simulink model "MATE_SynchronousMachineV2"  (R2024b)
settings: Solver=FixedStepDiscrete  StartTime=0.0  StopTime=6  FixedStep=Ts  RelTol=1e-4  EnableMultiTasking=on
PostLoadFcn:
  | Ts=25e-6;offset=4;
InitFcn:
  | Ts=25e-6;offset=4;
undefined symbols (not defined in the file): DiscIntNeverNeededParam, MATE, Phase, Rsnu, Single
libraries: fl_lib x76, nesl_utility x59, ee_lib x14, artemis x9, simetran x5, powerlib_extras x3, simetranss x2, simulink_extras x2, simulink x2
(part 2 of 5)

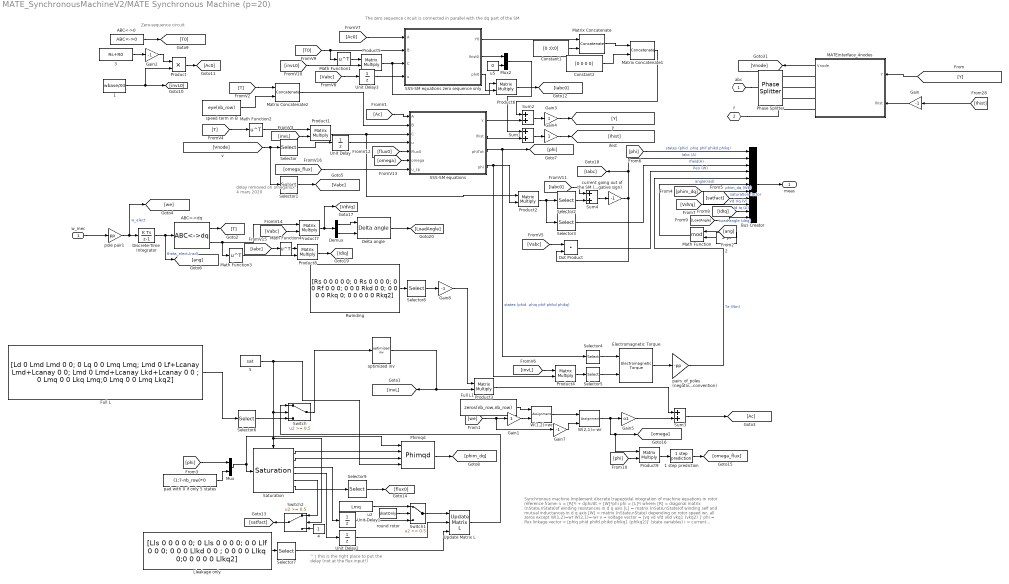
== system MATE_SynchronousMachineV2/MATE Synchronous Machine (p=20) ==
  note: delay removed
      | on omegaflux
      | 4 mars 2020
  note: Synchronous machine
      | Implement discrete trapezoidal integration of machine equations in rotor reference frame:
      |   v = [R]*i + dphi/dt + [W]*phi
      | phi = [L]*i
      |
      | where:
      | [R] = diagonal matrix (nState,nState)of winding resistances in d q axis
      | [L] = matrix (nSate,nState)of winding self and mutual inductances in d q axis
      | [W] = matrix (nState,nState) depending on rotor speed wr,
      |       all zeros except W(1,2)=wr  W(2,1)=-wr
      |
      |   v = voltage vector      = [vq   vd   vfd   vkd   vkq1   (vkq2)  ]'
      | phi = flux linkage vector = [phiq phid phifd phikd phikq1 (phikq2)]' (state variables)
      |   i = current vector      = [iq   id   ifd   ikd   ikq1   (ikq2)  ]'
      |
      | if RotorType=Salient-Pole, nState=5
      | if RotorType=Round,        nState=6
  note: ^
      | |
      | this is the right place to put the delay
      | (not at the flux input!)
  note: The zero sequence circuit is connected in parallel with the dq part of the SM
  note: Zero-sequence circuit
  w_mec : Inport
  1 : Constant  Value=wbase/X0
  1 step prediction : artemis/SSN/SSN rotating machines/SSN Synchronous Machine/1 step prediction  SystemSampleTime=-1  VariantActivationTime=update diagram  AllowFlexibleInterface=on  Latency=0  AutoFrameSizeCalculation=off
      settings: SourceProductName=Artemis
  2 : Constant  Value=2*pi
  3 : Constant  Value=Rs+R0
  4 : Constant
  5 : Constant  Value=sat
  ABC<->0 : artemis/SSN/SSN rotating machines/SSN Synchronous Machine/ABC<->0  SystemSampleTime=-1  VariantActivationTime=update diagram  AllowFlexibleInterface=on  Latency=0  AutoFrameSizeCalculation=off
      settings: SourceProductName=Artemis
  ABC<->dq : artemis/SSN/SSN rotating machines/SSN Synchronous Machine/ABC<->dq  SystemSampleTime=-1  VariantActivationTime=update diagram  AllowFlexibleInterface=on  Latency=0  AutoFrameSizeCalculation=off
      settings: SourceProductName=Artemis
  Bus Creator : BusCreator  Inputs=11
  Constant1 : Constant  Value=[0 ;0;0]  VectorParams1D=off
  Constant2 : Constant  Value=[0 0 0 0]  VectorParams1D=off
  Delta angle : artemis/SSN/SSN rotating machines/SSN Synchronous Machine/Delta angle  SystemSampleTime=-1  VariantActivationTime=update diagram  AllowFlexibleInterface=on  Latency=0  AutoFrameSizeCalculation=off
      settings: SourceProductName=Artemis
  Demux : Demux  Outputs=2
  Discrete-Time Integrator : DiscreteIntegrator  InitialCondition=theta_0  SampleTime=Ts  ICPrevOutput=DiscIntNeverNeededParam  ICPrevScaledInput=DiscIntNeverNeededParam
  Dot Product : DotProduct  OutDataTypeStr=Inherit: Inherit via internal rule
  Electromagnetic Torque : artemis/SSN/SSN rotating machines/SSN Synchronous Machine/Electromagnetic Torque  SystemSampleTime=-1  VariantActivationTime=update diagram  AllowFlexibleInterface=on  Latency=0  AutoFrameSizeCalculation=off
      settings: SourceProductName=Artemis
  Full L : Constant  Value="[Ld 0 Lmd Lmd 0 0; 0 Lq 0 0  Lmq Lmq; Lmd 0 Lf+Lcanay Lmd+Lcanay 0 0; Lmd 0 Lmd+Lcanay Lkd+Lcanay 0 0 ; 0 Lmq 0 0 Lkq Lmq;0 Lmq 0 0 Lmq Lkq2]"
  Full L1 : Constant  Value=zeros(nb_row,nb_row)
  Gain : Gain  Gain=-1
  Gain1 : Gain  SaturateOnIntegerOverflow=on  OutDataTypeStr=Inherit: Same as input  ParamDataTypeStr=Inherit: Same as input
  Gain2 : Gain  Gain=-1
  Gain3 : Gain
  Gain4 : Gain
  Gain5 : Gain  Gain=o1
  Gain7 : Gain  Gain=-1  SaturateOnIntegerOverflow=on  OutDataTypeStr=Inherit: Same as input  ParamDataTypeStr=Inherit: Same as input
  Gain8 : Gain  Gain=-1
  Lleakage only : Constant  Value="[Lls 0 0 0 0 0; 0 Lls 0 0  0 0; 0 0 Llf 0 0 0; 0 0 0 Llkd 0 0 ; 0 0 0 0 Llkq 0;0 0 0 0 0 Llkq2]"
  MATEinterface_4nodes : Subsystem
  Math Function : Math  Operator=mod  SignedPower=on
  Math Function{1..4} (4 alike) : Math  Operator=transpose  SignedPower=on
  Matrix Concatenate : Concatenate  Mode=Multidimensional array  ConcatenateDimension=2
  Matrix Concatenate1 : Concatenate  Mode=Multidimensional array
  Matrix Concatenate2 : Concatenate  Mode=Multidimensional array  ConcatenateDimension=2
  Mux : Mux  Inputs=2
  Mux2 : Mux  Inputs=2
  Phase Splitter : ee_lib/Connectors & References/Phase Splitter
  Phimqd : artemis/SSN/SSN rotating machines/SSN Synchronous Machine/Phimqd  SystemSampleTime=-1  VariantActivationTime=update diagram  AllowFlexibleInterface=on  Latency=0  AutoFrameSizeCalculation=off
      settings: SourceProductName=Artemis
  Product : Product  RndMeth=Zero
  Product{1..9} (9 alike) : Product  Multiplication=Matrix(*)  SaturateOnIntegerOverflow=on  OutDataTypeStr=Inherit: Same as first input
  Rwinding : Constant  Value="[Rs 0 0 0 0 0; 0 Rs 0 0 0 0; 0 0 Rf  0 0 0; 0 0 0 Rkd 0 0; 0 0 0 0  Rkq 0; 0 0 0 0 0 Rkq2]"
  SSS-SM equations : Subsystem
  SSS-SM equations zero sequence only : Subsystem
  Saturation : artemis/SSN/SSN rotating machines/SSN Synchronous Machine/Saturation  SystemSampleTime=-1  VariantActivationTime=update diagram  AllowFlexibleInterface=on  Latency=0  AutoFrameSizeCalculation=off
      settings: SourceProductName=Artemis
  Selector : Selector  InputPortWidth=4  IndexOptions=Index vector (dialog)  Indices=[1 2 3 4]  OutputSizes=1
  Selector1 : Selector  InputPortWidth=4  IndexOptions=Index vector (dialog)  Indices=[1 2 3 ]  OutputSizes=1
  Selector2 : Selector  InputPortWidth=4  IndexOptions=Index vector (dialog)  Indices=[1 2 3 ]  OutputSizes=1
  Selector3 : Selector  InputPortWidth=4  IndexOptions=Index vector (dialog)  Indices=[4 ]  OutputSizes=1
  Selector4 : Selector  InputPortWidth=nb_row  IndexOptions=Index vector (dialog)  Indices=[1 2]  OutputSizes=1
  Selector5 : Selector  InputPortWidth=nb_row  IndexOptions=Index vector (dialog)  Indices=[1 2]  OutputSizes=1
  Selector6 : Selector  NumberOfDimensions=2  InputPortWidth=3  IndexOptions=Index vector (dialog),Index vector (dialog)  Indices=[1:nb_row],[1:nb_row]  OutputSizes=1,1
  Selector7 : Selector  NumberOfDimensions=2  InputPortWidth=3  IndexOptions=Index vector (dialog),Index vector (dialog)  Indices=[1:nb_row],[1:nb_row]  OutputSizes=1,1
  Selector8 : Selector  NumberOfDimensions=2  InputPortWidth=3  IndexOptions=Index vector (dialog),Index vector (dialog)  Indices=[1:nb_row],[1:nb_row]  OutputSizes=1,1
  Selector9 : Selector  InputPortWidth=6  IndexOptions=Index vector (dialog)  Indices=[1:nb_row]  OutputSizes=1
  Sum{1..4} (4 alike) : Sum  SaturateOnIntegerOverflow=on
  Switch : Switch  Threshold=0.5  SaturateOnIntegerOverflow=off  InputSameDT=off
  Switch1 : Switch  Threshold=0.5  SaturateOnIntegerOverflow=off  InputSameDT=off
  Switch2 : Switch  Threshold=0.5  SaturateOnIntegerOverflow=off  InputSameDT=off
  Unit Delay : UnitDelay  SampleTime=Ts  HasFrameUpgradeWarning=on
  Unit Delay1 : UnitDelay  InitialCondition=Lmq  SampleTime=Ts  HasFrameUpgradeWarning=on
  Unit Delay2 : UnitDelay  InitialCondition=Lmd  SampleTime=Ts  HasFrameUpgradeWarning=on
  Unit Delay3 : UnitDelay  SampleTime=Ts  HasFrameUpgradeWarning=on
  Update Matrix L : artemis/SSN/SSN rotating machines/SSN Synchronous Machine/Update Matrix L  SystemSampleTime=-1  VariantActivationTime=update diagram  AllowFlexibleInterface=on  Latency=0  AutoFrameSizeCalculation=off
      settings: SourceProductName=Artemis
  W(1,2)=wr : Assignment  NumberOfDimensions=2  IndexOptions=Index vector (dialog),Index vector (dialog)  Indices=1,2  OutputSizes=1,1
  W(2,1)=-wr : Assignment  NumberOfDimensions=2  IndexOptions=Index vector (dialog),Index vector (dialog)  Indices=2,1  OutputSizes=1,1
  current going out of the SM (negative sign) : Gain  Gain=-1
  optimized inv : artemis/SSN/SSN rotating machines/SSN Synchronous Machine/optimized inv  SystemSampleTime=-1  VariantActivationTime=update diagram  AllowFlexibleInterface=on  Latency=0  AutoFrameSizeCalculation=off
      settings: SourceProductName=Artemis
  pad with 0 if only 5 states : Constant  Value=(1:7-nb_row)*0
  pairs_of_poles (negative sign for generator convention) : Gain  Gain=-pp
  pole pair1 : Gain  Gain=pp
  round rotor : Constant  Value=dsatOnly
  speed term in B : Constant  Value=eye(nb_row)  VectorParams1D=off
  u2 : Constant  Value=Lmq
  u5 : Constant  Value=0
  "abc   " : PMIOPort  Side=Right
  f : PMIOPort  Port=2  Side=Left
  meas : Outport  VectorParamsAs1DForOutWhenUnconnected=off
  wires:
  [Ihist] -> Gain/1
  Constant1/1 -> Matrix Concatenate/2
  Lleakage only/1 -> Selector7/1
  Delta angle/1 -> [LoadAngle]
  Gain7/1 -> W(2,1)=-wr/2
  Matrix Concatenate1/1 -> Sum2/1
  [phi] -> Product9/2
  W(1,2)=wr/1 -> W(2,1)=-wr/1
  Product2/1 -> Selector2/1, Selector3/1
  Selector2/1 -> Sum4/2
  Unit Delay/1 -> SSS-SM equations/4(u)
  [Vabc] -> Product7/2
  [invL] -> Product1/2
  [omega] -> SSS-SM equations/6(omega)
  SSS-SM equations zero sequence only/3(phi0) -> Product6/2
  ABC<->dq/1 -> [T]
  SSS-SM equations/1(Y) -> Sum2/2
  [Vabc] -> Unit Delay3/1
  w_mec/1 -> pole pair1/1
  3/1 -> Gain2/1
  [IdIq] -> Bus Creator/10  "Id Iq (A)"
  Selector3/1 -> Bus Creator/3  "Ifield(A)"
  Matrix Concatenate2/1 -> SSS-SM equations/2(B)
  [Iabc] -> Math Function4/1
  current going out of the SM (negative sign)/1 -> Dot Product/2, Bus Creator/2, [Iabc]  "Iabc (A)"
  [T] -> Matrix Concatenate2/1
  1/1 -> Product/2, [invL0]
  Saturation/1 -> Phimqd/2
  Math Function1/1 -> Product5/1
  speed term in B/1 -> Matrix Concatenate2/2
  u5/1 -> Mux2/2
  u2/1 -> Switch1/1
  Selector8/1 -> Gain8/1
  [VdVq] -> Bus Creator/9  "Vd Vq (V)"
  Selector9/1 -> [flux0]
  Product4/1 -> Selector5/1
  Math Function3/1 -> Product8/2
  pad with 0 if only 5 states/1 -> Mux/2
  2/1 -> Math Function/2
  Mux/1 -> Phimqd/1, Saturation/1
  Product/1 -> [Ac0]
  SSS-SM equations/2(Ihist) -> Sum1/2
  [Ac] -> SSS-SM equations/1(A)
  Product8/1 -> [IdIq]
  Dot Product/1 -> Bus Creator/4  "Peo (W)"
  [we] -> Gain7/1, Gain1/1
  Product6/1 -> [Iabc0]
  Switch1/1 -> Update Matrix L/1
  Rwinding/1 -> Selector8/1
  Gain3/1 -> [Y]
  [phi] -> Mux/1
  [invL0] -> Product5/2
  Sum2/1 -> Gain3/1
  optimized inv/1 -> [invL], Product3/2
  [Iabc0] -> Sum4/1
  [Ac0] -> SSS-SM equations zero sequence only/1(A)
  Selector6/1 -> Switch/3
  Gain1/1 -> W(1,2)=wr/2
  Selector1/1 -> [Vabc]
  1 step prediction/1 -> [omega_flux]
  ABC<->dq/2 -> Math Function3/1, Product7/1
  Mux2/1 -> Sum1/1
  SSS-SM equations/4(phi) -> Product4/2, Product2/2
  [satfact] -> Bus Creator/8  "saturation factor"
  Full L1/1 -> W(1,2)=wr/1
  Full L/1 -> Selector6/1
  Selector/1 -> Unit Delay/1
  Switch/1 -> optimized inv/1
  [Vabc] -> Dot Product/1
  W(2,1)=-wr/1 -> Gain5/1, [omega], Product9/1
  Demux/2 -> Delta angle/2
  Product5/1 -> SSS-SM equations zero sequence only/3(C), Product6/1
  5/1 -> Switch2/2, Saturation/Enable, Switch/2, Phimqd/4
  Saturation/4 -> Unit Delay2/1
  Gain5/1 -> Sum3/2
  pairs_of_poles (negative sign for generator convention)/1 -> Bus Creator/5  "Te (Nm)"
  Bus Creator/1 -> meas/1
  [Vnode] -> Selector/1, Selector1/1
  [T0] -> SSS-SM equations zero sequence only/2(B), Math Function1/1
  Sum1/1 -> Gain4/1
  SSS-SM equations zero sequence only/2(Ihist0) -> Mux2/1
  Gain2/1 -> Product/1
  Phimqd/1 -> [phim_dq]
  Unit Delay3/1 -> SSS-SM equations zero sequence only/4(u)
  SSS-SM equations zero sequence only/1(Y0) -> Matrix Concatenate/1
  [flux0] -> SSS-SM equations/5(Flux0)
  Demux/1 -> Delta angle/1
  Constant2/1 -> Matrix Concatenate1/2
  Gain8/1 -> Product3/1
  round rotor/1 -> Switch1/2
  Math Function2/1 -> Product1/1
  Switch2/1 -> [satfact]
  Update Matrix L/1 -> Switch/1
  Product1/1 -> SSS-SM equations/3(C), Product2/1
  SSS-SM equations/3(phiTot) -> Selector4/1, [phi]  "states (phid  phiq phif phikd phikq)"
  4/1 -> Switch2/3
  Sum3/1 -> [Ac]
  [T] -> Math Function2/1
  Selector7/1 -> Update Matrix L/3
  Product9/1 -> 1 step prediction/1
  Saturation/2 -> Phimqd/3
  Product3/1 -> Sum3/1
  Saturation/3 -> Unit Delay1/1
  Discrete-Time Integrator/1 -> [ang], ABC<->dq/1  "theta_elect (rad)"
  ABC<->0/1 -> [T0]
  Math Function/1 -> Bus Creator/6  "angle(rad)"
  pole pair1/1 -> Discrete-Time Integrator/1, [we]  "w_elect"
  Gain4/1 -> [Ihist]
  Unit Delay2/1 -> Update Matrix L/2
  Saturation/6 -> Selector9/1
  Electromagnetic Torque/1 -> pairs_of_poles (negative sign for generator convention)/1
  Math Function4/1 -> Product8/1
  [ang] -> Math Function/1
  [phi] -> Bus Creator/1  "states (phid  phiq phif phikd phikq)"
  Matrix Concatenate/1 -> Matrix Concatenate1/1
  [invL] -> Product4/1
  Unit Delay1/1 -> Switch1/3
  Selector4/1 -> Electromagnetic Torque/1
  Saturation/5 -> Switch2/1
  Product7/1 -> [VdVq], Demux/1
  [omega_flux] -> SSS-SM equations/7(u_sp)
  [phim_dq] -> Bus Creator/7  "phim_dq (Wb)"
  [LoadAngle] -> Bus Creator/11  "Load angle (deg)"
  Selector5/1 -> Electromagnetic Torque/2
  Sum4/1 -> current going out of the SM (negative sign)/1
  MATEinterface_4nodes/1(Vnode) -> [Vnode]
  [Y] -> MATEinterface_4nodes/1(Y)
  Gain/1 -> MATEinterface_4nodes/2(Ihist)
  connections:
  "abc   "/RConn1 -- Phase Splitter/LConn1
  MATEinterface_4nodes/RConn1 -- Phase Splitter/RConn1
  MATEinterface_4nodes/RConn2 -- Phase Splitter/RConn2
  MATEinterface_4nodes/RConn3 -- Phase Splitter/RConn3
  f/RConn1 -- MATEinterface_4nodes/RConn4

== system MATE_SynchronousMachineV2/MATE_LineCommutatedConverter ==
  g : Inport
  MATEPREP : Subsystem  Commented=on
  MATE_AGGREG : Subsystem
  Phase Splitter2 : ee_lib/Connectors & References/Phase Splitter
  abc : PMIOPort  Side=Left
  + : PMIOPort  Port=2  Side=Right
  - : PMIOPort  Port=3  Side=Right
  meas : Outport
  wires:
  g/1 -> MATEPREP/1(g), MATE_AGGREG/1(g)
  MATE_AGGREG/1(meas) -> meas/1
  connections:
  MATEPREP/RConn2 -- MATE_AGGREG/RConn2 -- -/RConn1
  MATEPREP/RConn1 -- MATE_AGGREG/RConn1 -- +/RConn1
  Phase Splitter2/RConn1 -- MATEPREP/LConn1 -- MATE_AGGREG/LConn1
  Phase Splitter2/RConn2 -- MATEPREP/LConn2 -- MATE_AGGREG/LConn2
  Phase Splitter2/RConn3 -- MATEPREP/LConn3 -- MATE_AGGREG/LConn3
  abc/RConn1 -- Phase Splitter2/LConn1

== system MATE_SynchronousMachineV2/Mesure et visualisation ==
  Discrete Mean value : Subsystem  mask(Discrete Mean value){Freq=60, Vinit=0, Ts=Ts}
      mask prompts: Freq "Fundamental frequency (Hz):"; Vinit "Initial input (DC component):"; Ts "Sample time:"
      mask help: Compute the mean value of the input signal over a running window of one cycle of the specified fundamental frequency.
      mask init:
      | SamplesPerCycle=1/Freq/Ts;
      | RoundSamplesPerCycle=ceil(SamplesPerCycle);
      | Delay=RoundSamplesPerCycle*Ts;
      | Corr1=(SamplesPerCycle-RoundSamplesPerCycle)/2;
      | Corr2=(SamplesPerCycle-RoundSamplesPerCycle)/SamplesPerCycle;
      | K1=Corr1*Corr2;
      | K2=Corr2 + Corr1*Corr2;
      mask Display: disp('Mean\n(discrete)')
  Mux : Mux  Inputs=2
  Mux3 : Mux  Inputs=2
  Mux4 : Mux  Inputs=2
  V1 Vref : Outport
  If IIfref : Outport  Port=2
  Vcc : Outport  Port=3
  wires:
  Discrete Mean value/1(Mean) -> Mux/2
  [Ucc] -> Mux/1, Discrete Mean value/1(In)
  Mux/1 -> Vcc/1  "Vcc - Vcc moyen (V)"
  [If] -> Mux3/1
  [Ifref] -> Mux3/2
  Mux3/1 -> If IIfref/1
  [V1] -> Mux4/1
  [Vref] -> Mux4/2
  Mux4/1 -> V1 Vref/1

== system MATE_SynchronousMachineV2/Model Initialization ==

== system MATE_SynchronousMachineV2/PQ ==
  note: 1) P = Va*Ia + Vb*Ib + Vc*Ic
  note: 2) Q = 1/sqrt(3)* (Vbc*Ia + Vca*Ib + Vab*Ic)
  note: This block computes the 3-phase instantaneous real power and reactive power using the following equations:
  note: Note: Equation 2 is valid only for a balanced and harmonic-free system.
  Vabc : Inport  PortDimensions=3
  Iabc : Inport  Port=2  PortDimensions=3
  Demux : Demux  Outputs=3
      settings: DisplayOption=none
  Mux : Mux  Inputs=3
  Mux1 : Mux  Inputs=2
  Product1 : Product  InputSameDT=on  SaturateOnIntegerOverflow=on  OutDataTypeStr=Inherit: Same as first input
  Product3 : Product  InputSameDT=on  SaturateOnIntegerOverflow=on  OutDataTypeStr=Inherit: Same as first input
  Sum : Sum  Inputs=+-  InputSameDT=on  SaturateOnIntegerOverflow=on  OutDataTypeStr=Inherit: Same as first input
  Sum1 : Sum  Inputs=1  InputSameDT=on  SaturateOnIntegerOverflow=on  OutDataTypeStr=Inherit: Same as first input
  Sum4 : Sum  Inputs=1  InputSameDT=on  SaturateOnIntegerOverflow=on  OutDataTypeStr=Inherit: Same as first input
  Sum5 : Sum  Inputs=+-  InputSameDT=on  SaturateOnIntegerOverflow=on  OutDataTypeStr=Inherit: Same as first input
  Sum6 : Sum  Inputs=+-  InputSameDT=on  SaturateOnIntegerOverflow=on  OutDataTypeStr=Inherit: Same as first input
  pu->V : Gain  Gain=1/sqrt(3)  SaturateOnIntegerOverflow=on  OutDataTypeStr=Inherit: Same as input  ParamDataTypeStr=Inherit: Same as input
  PQ : Outport  VectorParamsAs1DForOutWhenUnconnected=off
  wires:
  Sum1/1 -> pu->V/1
  Product3/1 -> Sum1/1
  Product1/1 -> Sum4/1
  Vabc/1 -> Product1/1, Demux/1
  Iabc/1 -> Product1/2, Product3/2
  Sum4/1 -> Mux1/1  "P"
  Demux/1 -> Sum/1, Sum6/2
  Demux/2 -> Sum/2, Sum5/1
  Demux/3 -> Sum5/2, Sum6/1
  Sum/1 -> Mux/3
  Sum5/1 -> Mux/1
  Sum6/1 -> Mux/2
  Mux/1 -> Product3/1
  pu->V/1 -> Mux1/2  "Q"
  Mux1/1 -> PQ/1

== system MATE_SynchronousMachineV2/turbine1 ==
  feild : Inport
  Te : Inport  Port=2
  Peo : Inport  Port=3
  Gain : Gain  Gain=1/(2*pi*60/20)
  Gain1 : Gain  Gain=1/202e6
  Gain3 : Gain  Gain=202e6
  Gain4 : Gain  Gain=1/(2*pi*60/20)
  Hydraulic Turbine and Governor : Subsystem  mask(Hydraulic Turbine and Governor){sm=[ 10/3  0.07 ], gate=[  0.01  0.97518  -0.1  0.1 ], reg=[  0.05  1.163  0.105  0  0.01  ], hyd=[  0  2.67  ], dref=0, po=0.802}
      mask prompts: sm "Servo-motor [ Ka()  Ta(sec) ]:"; gate "Gate opening limits [ gmin,gmax(pu)    vgmin,vgmax(pu/s) ]:"; reg "Permanent droop and regulator  [ Rp() Kp() Ki() Kd() Td(s) ]:"; hyd "Hydraulic turbine [ beta()  Tw(sec) ]:"; dref "Droop reference (0=power error, 1=gate opening):"; po "Initial mechanical power (pu):"
      mask help: Implements a hydraulic turbine combined to a PID governor system.
      mask init:
      | %block = gcb;
      | %[Ts, WantBlockChoice,ka,ta,gmin,gmax,vgmin,vgmax,Rp,Kp,ki,kd,td,beta,tw,go] = powericon('HydraulicTurbineInit',block,sm,gate,reg,hyd,po);
      | ka =sm (1 ); 
      | ta =sm (2 ); 
      | gmin =gate (1 ); 
      | gmax =gate (2 ); 
      | vgmin =gate (3 ); 
      | vgmax =gate (4 ); 
      | Rp =reg (1 ); 
      | kp =reg (2 ); 
      | ki =reg (3 ); 
      | kd =reg (4 ); 
      | td =reg (5 ); 
      | beta =hyd (1 ); 
      | tw =hyd (2 ); 
      | go =po *(gmax -gmin ); 
      | %powericon('SetInternalModels','set',block,WantBlockChoice);
      settings: OpenFcn=sps_rtmsupport('OpenFcn',gcbh)
      mask Help: helpview(psbhelp);
      mask Display: disp('')
  Mechanical model : Subsystem  mask(Synchronous machine mechanical model){J=3.4111e+06, F=0, fo=60/20, Ts=Ts}
      mask prompts: J "Inertia (kg.m^2)"; F "Friction (N.n.s)"; fo "Initial mechanical frequency (Hz)"; Ts "Sample Time (s)"
      mask help:
      | This is the mechanical equation of a synchronous machine.
      |
      | all values in SI.
      | J: inertia
      | F:friction
      | Te: torque input from the SM
      | Pin: power from the turbine
      | wmec: mechanical speed of the SM.
      | delta_wm: speed deviation
  Pref : Constant  Value=0.8
  Product1 : Product
  Terminator : Terminator
  wref : Constant
  w : Outport
  wires:
  Hydraulic Turbine and Governor/2(gate) -> Terminator/1
  Hydraulic Turbine and Governor/1(Pm) -> Gain3/1
  Gain1/1 -> Hydraulic Turbine and Governor/4(Pe0)
  Gain/1 -> Hydraulic Turbine and Governor/3(we)
  wref/1 -> Hydraulic Turbine and Governor/1(wref)
  Mechanical model/2(delta_wm) -> Gain4/1
  Pref/1 -> Product1/2
  Product1/1 -> Hydraulic Turbine and Governor/2(Pref)
  Gain3/1 -> Mechanical model/2(Pin)
  Mechanical model/1(wmec) -> Gain/1, w/1
  Gain4/1 -> Hydraulic Turbine and Governor/5(dw)
  feild/1 -> Product1/1
  Te/1 -> Mechanical model/1(Te)
  Peo/1 -> Gain1/1

== system MATE_SynchronousMachineV2/Command/Regulateur de courant ==
  If (pu) : Inport
  If_ref : Inport  Port=2
  Discrete 1st-Order Filter : Subsystem  mask(Discrete 1st-Order Filter){FilterType=Lowpass, Tc=1e-3, Ts=Ts, Initialize=off, Vac_Init=[0, 0, 60], Vdc_Init=0, PlotResponse=off, param1=[1 500 0.1]}
      mask prompts: FilterType "Filter Type:"; Tc "Time constant (s):"; Ts "Sample time:"; Initialize "Initialize filter states"; Vac_Init "AC initial input: [ Mag  Phase(degrees)  Freq(Hz) ]"; Vdc_Init "DC Initial input:"; PlotResponse "Plot filter response"; param1 "Frequency range(Hz) : [Start  End  Inc.]"
      mask init:
      | switch FilterType
      | case 1, % Lowpass
      |     X=[0 1 2 3 4];
      |     Y=[-2 -2 -3 -4 -4];
      |     numc=1;
      |     denc=[Tc 1];
      | case 2,   % Highpass
      |     X=[0 1 2 3 4];
      |     Y=[-4 -4 -3 -2 -2];
      |     numc=[1 0];
      |     denc=[1 1/Tc];
      | end
      | %
      | [Ac,Bc,Cc,Dc]=tf2ss(numc,denc);
      | %
      | %  Conversion to discrete transfer function
      | nstates = size(Ac,1);
      | if Ts<=0
      |     message = 'The Sample time parameter must be greater than zero. Note that specifying inherited sample time (-1) does not work for this block';
      |     error(message);
      | end
      | invexp = inv(eye(nstates) - (Ts/2)*Ac);
      | Ad = invexp*(eye(nstates) + (Ts/2)*Ac);
      | Bd = invexp*Bc;
      | Cd = Cc*invexp*Ts;
      | Dd = Cc*invexp*Bc*(Ts/2) + Dc;
      | %
      | if Initialize==1  % Compute initial conditions on states
      |     u1=Vac_Init(1)*exp(j*Vac_Init(2)*pi/180);
      |     u2=Vdc_Init*exp(j*90*pi/180);
      |     u=u1+u2;
      |     u0=imag(u); % input at  t=0;
      |     I=eye(size(Ac));
      |     sI1=I*j*(2*pi*Vac_Init(3));
      |     sI2=I*j*0;
      |     x=inv(sI1-Ac)*Bc*u1 + inv(sI2-Ac)*Bc*u2;
      |     x0c=imag(x);
      |     x0d=(I-Ac*Ts/2)*x0c/Ts - Bc/2*u0;
      | else
      |     x0d=0;
      | end
      | 
      | %
      | if PlotResponse==1 % Plot frequency and step response
      | t=[0:Tc/1000:7*Tc];
      | f=param1(1):param1(3):param1(2);
      | w=2*pi*f;
      | switch FilterType
      | 	case 1, % Lowpass
      | 		Ystep=1 - exp(-t/Tc);
      | 		RepFreq=1./(1+Tc*j.*w);
      | 	case 2,   % Highpass
      | 		Ystep=exp(-t/Tc);
      | 		RepFreq=1./(1 + (1./(Tc*j.*w)));
      | end
      | %
      | Mag=abs(RepFreq);
      | Pha=angle(RepFreq)*180/pi;
      | %
      | figure(1)
      | subplot(2,1,1)
      | plot(f,Mag)
      | grid
      | title('Bode Diagram')
      | ylabel('Magnitude')
      | subplot(2,1,2)
      | plot(f,Pha)
      | ylabel('Phase (deg)')
      | xlabel('Frequency (Hz)')
      | grid
      | figure(2)
      | plot(t,Ystep)
      | grid
      | ylabel('Amplitude')
      | xlabel('Time (s)')
      | title('Step Response')
      | end
      mask TypeOptions FilterType: Lowpass | Highpass
      mask Display: plot(X,Y);
  Discrete PI Controller1 : Subsystem  mask(Discrete PI Controller){Kp=400, Ki=1000, Par_Limits=[150 10], Init=79, Ts=Ts}
      mask prompts: Kp "Proportional gain (Kp):"; Ki "Integral gain (Ki):"; Par_Limits "Output limits: [ Upper   Lower ]"; Init "Output initial value:"; Ts "Sample time:"
      mask help: This block implements a basic discrete PI controller.
      mask init:
      | UpperLimit=Par_Limits(1);
      | LowerLimit=Par_Limits(2);
      mask Display: disp('PI');
  Sum : Sum  Inputs=|+-
  alpha : Outport
  wires:
  Discrete 1st-Order Filter/1(Out) -> Sum/1
  If (pu)/1 -> Discrete 1st-Order Filter/1(In)
  If_ref/1 -> Sum/2
  Sum/1 -> Discrete PI Controller1/1(Error)
  Discrete PI Controller1/1(Out) -> alpha/1

== system MATE_SynchronousMachineV2/Command/Regulateur de tension (Mode automatique) ==
  note: Regulateur de tension
  Vabc (pu) : Inport
  Vref : Inport  Port=2
  Discrete PI Controller1 : Subsystem  mask(Discrete PI Controller){Kp=Kp_V, Ki=Ki_V, Par_Limits=[2.46 0.33], Init=1, Ts=Ts}
      mask prompts: Kp "Proportional gain (Kp):"; Ki "Integral gain (Ki):"; Par_Limits "Output limits: [ Upper   Lower ]"; Init "Output initial value:"; Ts "Sample time:"
      mask help: This block implements a basic discrete PI controller.
      mask init:
      | UpperLimit=Par_Limits(1);
      | LowerLimit=Par_Limits(2);
      mask Display: disp('PI');
  Discrete 3-phase Positive-Sequence Fundamental Value : Subsystem  mask(Discrete 3-phase Positive-sequence fundamental value){Freq=60, Par_Init=[0 0], Ts=Ts}
      mask prompts: Freq "Fundamental frequency (Hz):"; Par_Init "Initial input (positive component): [ Mag  Phase(degrees) ]"; Ts "Sample time:"
      mask help: Compute the positive-sequence component of the input signal at the given fundamental frequency. The input is set of three balanced or unbalanced signals which may contain harmonics.
      mask init:
      | SamplesPerCycle=1/Freq/Ts;
      | RoundSamplesPerCycle=round(SamplesPerCycle);
      | Delay=RoundSamplesPerCycle*Ts - Ts/2;
      | Correction=SamplesPerCycle/RoundSamplesPerCycle - 1;
      | Real_Init=Par_Init(1)*cos(pi/180*Par_Init(2));
      | Imag_Init=Par_Init(1)*sin(pi/180*Par_Init(2));
      mask Display: disp('')
  Sum : Sum  Inputs=|-+
  Terminator : Terminator
  Iref : Outport
  tag scope: V1=global, Vref=global
  wires:
  Discrete 3-phase Positive-Sequence Fundamental Value/2(Phase) -> Terminator/1
  Vabc (pu)/1 -> Discrete 3-phase Positive-Sequence Fundamental Value/1(abc)
  Discrete PI Controller1/1(Out) -> Iref/1
  Sum/1 -> Discrete PI Controller1/1(Error)
  Vref/1 -> Sum/2, [Vref]
  Discrete 3-phase Positive-Sequence Fundamental Value/1(Mag) -> Sum/1, [V1]

== system MATE_SynchronousMachineV2/Command/Synchro Generateur d'mpulsions  ==
  Vabc_138 (pu) : Inport
  alpha(deg) : Inport  Port=2
  Demux : Demux  Outputs=3
  Discrete 3-phase PLL : Subsystem  mask(Discrete 3-phase PLL){Fmin=45, Par_Init=[0 60], ParK=[ 180 3200 1 ], Ts=Ts, AGC=on}
      mask prompts: Fmin "Minimum frequency (Hz):"; Par_Init "Initial inputs:[ Phase(degrees)   Frequency(Hz) ]"; ParK "Regulator gains [ Kp  Ki  Kd ]"; Ts "Sample time:"; AGC "Enable Automatic Gain Control"
      mask help:
      | This Phase Locked Loop (PLL) system can be used  to synchronize on a set of variable frequency, three-phase sinusoidal signals. If the Automatic Gain Control is enabled, the input (phase error) of the PLL regulator is scaled according to the input signals magnitude.
      |
      | For optimal performance, the following settings are recommended:
      |   [ Kp Ki  Kd ] = [ 180  3200  1 ]
      |   "Enable Automatic Gain Control" checked
      |
      | Input 1: Vector containing the normalized three-phase signals [Va Vb Vc]
      | Output 1:  Measured frequency (Hz) = w/(2pi)
      | Output 2:  Ramp w.t varying between  0 and 2*pi,
      |      synchronized on zero crossings of the fundamental (positive-sequence) of phase A.
      | Output 3: Vector [sin(wt) cos(wt)]
      mask init:
      | Kp=ParK(1);
      | Ki=ParK(2);
      | if length(ParK)==2
      |     Kd=0;
      | else
      |     Kd=ParK(3);
      | end    
      | Phase_Init=Par_Init(1);
      | Finit=Par_Init(2);
      settings: OpenFcn=power_openblockproxy();
      mask Display: disp('')
  Discrete Synchronized 12-Pulse Generator : Subsystem  mask(Discrete synchronized 12-pulse generator){Delta=D1 (lagging), pwidth=20, Double_Pulse=on, Ts=Ts}
      mask prompts: Delta "Delta winding connection"; pwidth "Pulse width (degrees)"; Double_Pulse "Double pulsing"; Ts "Sample time"
      mask help:
      | Use this block to fire the 12 thyristors of a 12-pulse converter.
      | Outputs 1 and 2 are two vectors of 6 pulses (0-1) to be sent to the two 6-pulse half bridges connected respectively to the Wye(Y) and Delta (D1 or D11) connected windings of the YYD converter transformer.
      | Pulses are individually synchronized on the 6 commutation voltages and generated alpha degrees after the increasing zero-crossings of the commutation voltages. The D pulses are either lagging or leading the Y pulses by 30 degrees.
      |
      | Input 'alpha_deg' :  Alpha firing signal (degrees).
      | Inputs 'A,B,C' : Phase-to-ground synchronization voltages  measured at the  primary side of the converter transformer.
      | Input 'Freq' : Frequency of the synchronization voltages (use a constant or the Freq PLL output)
      | Input 'Block' allows  blocking of the pulses when the applied signal is non zero.
      |
      | When the 'Douple pulsing' option is checked, two pulses are sent to each thyristor: a 1st pulse when the alpha angle is reached, then a 2nd pulse 60 degrees later, when the next thyristor is fired.
      mask init:
      | if (Delta == 1)
      |     D1 = 1;
      | else
      |     D1 = 0;
      | end
      mask TypeOptions Delta: D1 (lagging) | D11 (leading)
      mask Display: plot(0,0,100,100,[80 62 62 47 47 30],[40 40 60 60 40 40]-5)
  Ground2 : Ground
  Terminator : Terminator
  Terminator1 : Terminator
  Terminator2 : Terminator
  P : Outport
  wires:
  Vabc_138 (pu)/1 -> Discrete 3-phase PLL/1(Vabc(pu)), Demux/1
  Ground2/1 -> Discrete Synchronized 12-Pulse Generator/6(Block)
  alpha(deg)/1 -> Discrete Synchronized 12-Pulse Generator/1(alpha_deg)
  Demux/1 -> Discrete Synchronized 12-Pulse Generator/2(A)
  Demux/2 -> Discrete Synchronized 12-Pulse Generator/3(B)
  Demux/3 -> Discrete Synchronized 12-Pulse Generator/4(C)
  Discrete 3-phase PLL/1(Freq) -> Discrete Synchronized 12-Pulse Generator/5(Freq)
  Discrete Synchronized 12-Pulse Generator/2(PD) -> P/1
  Discrete 3-phase PLL/2(wt) -> Terminator/1
  Discrete 3-phase PLL/3(Sin_Cos) -> Terminator1/1
  Discrete Synchronized 12-Pulse Generator/1(PY) -> Terminator2/1

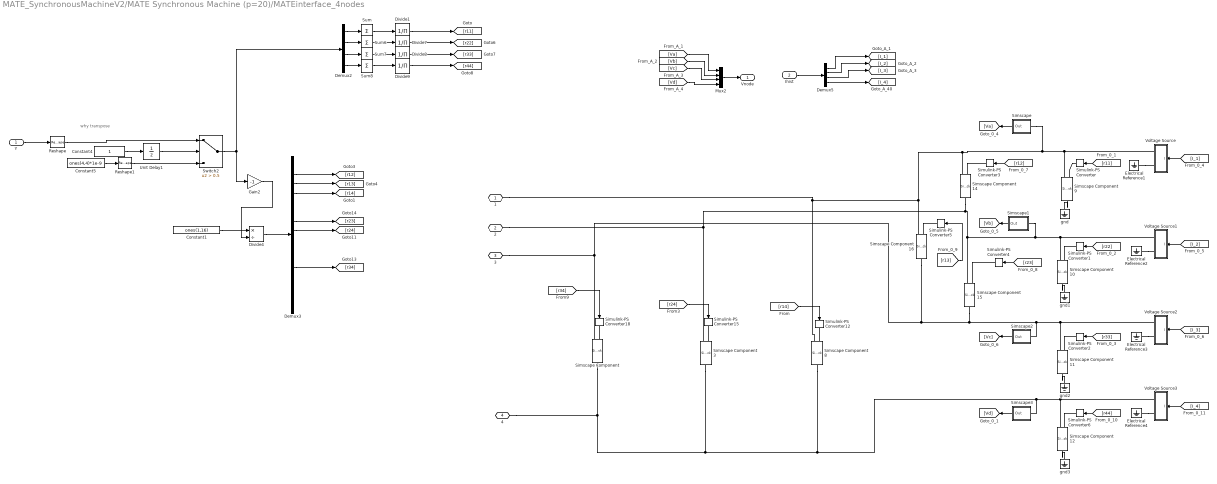
== system MATE_SynchronousMachineV2/MATE Synchronous Machine (p=20)/MATEinterface_4nodes ==
  note: why transpose
  Y : Inport
  Ihist : Inport  Port=2
  Constant1 : Constant  Value=ones(1,16)
  Constant4 : Constant
  Constant5 : Constant  Value=ones(4,4)*1e-9
  Demux2 : Demux  Outputs=[4 4 4 4]
      settings: DisplayOption=none
  Demux3 : Demux  Outputs=16
      settings: DisplayOption=none
  Demux5 : Demux  Outputs=[1 1 1 1 ]
      settings: DisplayOption=none
  Divide{1,7..9} (4 alike) : Product  Inputs=/
  Divide4 : Product  Inputs=*/  CollapseMode=Specified dimension
  Electrical Reference{1..4} (4 alike) : fl_lib/Electrical/Electrical Elements/Electrical Reference
  Gain2 : Gain  Gain=-1
  Mux2 : Mux  Inputs=[1 1 1 1 ]
  Reshape : Reshape
  Reshape1 : Reshape
  Simscape : Subsystem
      mask Display: disp('V')
  Simscape Component{,3,8..12,14..16} (10 alike) : SimscapeComponentBlock  SourceFile=variable_resistor_unlimited  ComponentPath=variable_resistor_unlimited  ComponentVariants="[\"variable_resistor_unlimited\"]"  ComponentVariantNames="[\"variable_resistor_unlimited\"]"  ClassName=variable_resistor_unlimited  SchemaVersion=1  R0=0 Ohm  Rmaxp=1e9 Ohm  Rmaxn=-1e9 Ohm  Rminp=1e-9 Ohm  Rminn=-1e-9 Ohm  i_specify=off  i_priority=None  i=0 A  i_nominal_specify=off  i_nominal_value=1  i_nominal_unit=A  v_specify=off  v_priority=None  v=0 V  v_nominal_specify=off  v_nominal_value=1  v_nominal_unit=V
      settings: CopyFcn=simscape.engine.sli.internal.componentblockcallback(gcbh,'COPY')  PreCopyFcn=simscape.engine.sli.internal.componentblockcallback(gcbh,'PRECOPY')  PreDeleteFcn=simscape.engine.sli.internal.componentblockcallback(gcbh,'PREDELETE')  InternalSimscapePortConfiguration="{\"Bottom\":[],\"Left\":[{\"id\":\"R\",\"label\":\"R\",\"type\":\"input\"},{\"id\":\"p\",\"label\":\"+\",\"type\":\"foundation.electrical.electrical\"}],\"Right\":[{\"id\":\"n\",\"label\":\"-\",\"type\":\"foundation.electrical.electrical\"}],\"Top\":[]}"
      mask Type: Variable Resistor
  Simscape1 : Subsystem
      mask Display: disp('V')
  Simscape2 : Subsystem
      mask Display: disp('V')
  Simscape3 : Subsystem
      mask Display: disp('V')
  Simulink-PS Converter{,1..6,12,15,18} (10 alike) : nesl_utility/Simulink-PS Converter  PhysicalDomain=network_engine_domain  SubClassName=ps_input  LeftPortType=input  RightPortType=output  PseudoPeriodic=off  Frequencies=[]  NoiseDistribution=none  NoiseParameters=[]  Unit=1  AffineConversion=off  FilteringAndDerivatives=provide  SimscapeFilterOrder=1  InputFilterTimeConstant=0.001  UdotUserProvided=0
  Sum{,6..8} (4 alike) : Sum  Inputs=+
  Switch2 : Switch  Criteria=u2 > Threshold  Threshold=0.5  SaturateOnIntegerOverflow=off  InputSameDT=off
  Unit Delay1 : UnitDelay  SampleTime=Ts  HasFrameUpgradeWarning=on
  Voltage Source : Subsystem
  Voltage Source1 : Subsystem
  Voltage Source2 : Subsystem
  Voltage Source3 : Subsystem
  gnd{,1..3} (4 alike) : fl_lib/Electrical/Electrical Elements/Electrical Reference
  1 : PMIOPort  Side=Right
  2 : PMIOPort  Port=2  Side=Right
  3 : PMIOPort  Port=3  Side=Right
  4 : PMIOPort  Port=4  Side=Right
  Vnode : Outport  VectorParamsAs1DForOutWhenUnconnected=off
  wires:
  [I_2] -> Voltage Source1/1(I)
  Simscape2/1(Out) -> [Vc]
  [I_3] -> Voltage Source2/1(I)
  Simscape/1(Out) -> [Va]
  Simscape1/1(Out) -> [Vb]
  [I_1] -> Voltage Source/1(I)
  Y/1 -> Reshape/1
  [r11] -> Simulink-PS Converter/1
  Sum/1 -> Divide1/1
  Divide1/1 -> [r11]
  [r22] -> Simulink-PS Converter1/1
  [r33] -> Simulink-PS Converter2/1
  [r12] -> Simulink-PS Converter3/1
  [r23] -> Simulink-PS Converter4/1
  [r13] -> Simulink-PS Converter5/1
  Demux2/1 -> Sum/1
  Divide7/1 -> [r22]
  Sum6/1 -> Divide7/1
  Demux2/2 -> Sum6/1
  Sum7/1 -> Divide8/1
  Divide8/1 -> [r33]
  Demux2/3 -> Sum7/1
  Demux2/4 -> Sum8/1
  Divide9/1 -> [r44]
  Sum8/1 -> Divide9/1
  [r44] -> Simulink-PS Converter6/1
  [I_4] -> Voltage Source3/1(I)
  Simscape3/1(Out) -> [Vd]
  [r14] -> Simulink-PS Converter12/1
  [r24] -> Simulink-PS Converter15/1
  Mux2/1 -> Vnode/1
  Ihist/1 -> Demux5/1
  Demux3/2 -> [r12]
  Demux3/3 -> [r13]
  Demux3/4 -> [r14]
  Constant1/1 -> Divide4/1
  [r34] -> Simulink-PS Converter18/1
  Reshape/1 -> Switch2/1
  Unit Delay1/1 -> Switch2/2
  Constant4/1 -> Unit Delay1/1
  Reshape1/1 -> Switch2/3
  Gain2/1 -> Divide4/2
  Demux5/4 -> [I_4]
  Demux5/3 -> [I_3]
  Demux5/2 -> [I_2]
  Demux5/1 -> [I_1]
  [Vd] -> Mux2/4
  [Vc] -> Mux2/3
  [Vb] -> Mux2/2
  [Va] -> Mux2/1
  Constant5/1 -> Reshape1/1
  Switch2/1 -> Demux2/1, Gain2/1
  Divide4/1 -> Demux3/1
  Demux3/7 -> [r23]
  Demux3/8 -> [r24]
  Demux3/12 -> [r34]
  connections:
  Simscape Component14/LConn2 -- Simscape Component9/LConn2 -- Voltage Source/RConn1 -- Simscape/LConn1 -- Simscape Component16/LConn2 -- 1/RConn1 -- Simscape Component8/LConn2
  Simscape Component11/LConn2 -- Voltage Source2/RConn1 -- Simscape2/LConn1 -- Simscape Component15/RConn1 -- Simscape Component16/RConn1 -- Simscape Component/LConn2 -- 3/RConn1
  Simscape Component10/LConn2 -- Voltage Source1/RConn1 -- Simscape1/LConn1 -- Simscape Component15/LConn2 -- Simscape Component14/RConn1 -- Simscape Component3/LConn2 -- 2/RConn1
  Electrical Reference2/LConn1 -- Voltage Source1/RConn2
  Electrical Reference3/LConn1 -- Voltage Source2/RConn2
  Electrical Reference1/LConn1 -- Voltage Source/RConn2
  Simscape Component9/RConn1 -- gnd/LConn1
  Simscape Component9/LConn1 -- Simulink-PS Converter/RConn1
  Simscape Component10/RConn1 -- gnd1/LConn1
  Simscape Component10/LConn1 -- Simulink-PS Converter1/RConn1
  Simscape Component11/RConn1 -- gnd2/LConn1
  Simscape Component11/LConn1 -- Simulink-PS Converter2/RConn1
  Simscape Component14/LConn1 -- Simulink-PS Converter3/RConn1
  Simscape Component15/LConn1 -- Simulink-PS Converter4/RConn1
  Simscape Component16/LConn1 -- Simulink-PS Converter5/RConn1
  4/RConn1 -- Simscape Component/RConn1 -- Simscape Component3/RConn1 -- Simscape Component8/RConn1 -- Simscape Component12/LConn2 -- Voltage Source3/RConn1 -- Simscape3/LConn1
  Simscape Component12/LConn1 -- Simulink-PS Converter6/RConn1
  Simscape Component12/RConn1 -- gnd3/LConn1
  Electrical Reference4/LConn1 -- Voltage Source3/RConn2
  Simscape Component8/LConn1 -- Simulink-PS Converter12/RConn1
  Simscape Component3/LConn1 -- Simulink-PS Converter15/RConn1
  Simscape Component/LConn1 -- Simulink-PS Converter18/RConn1

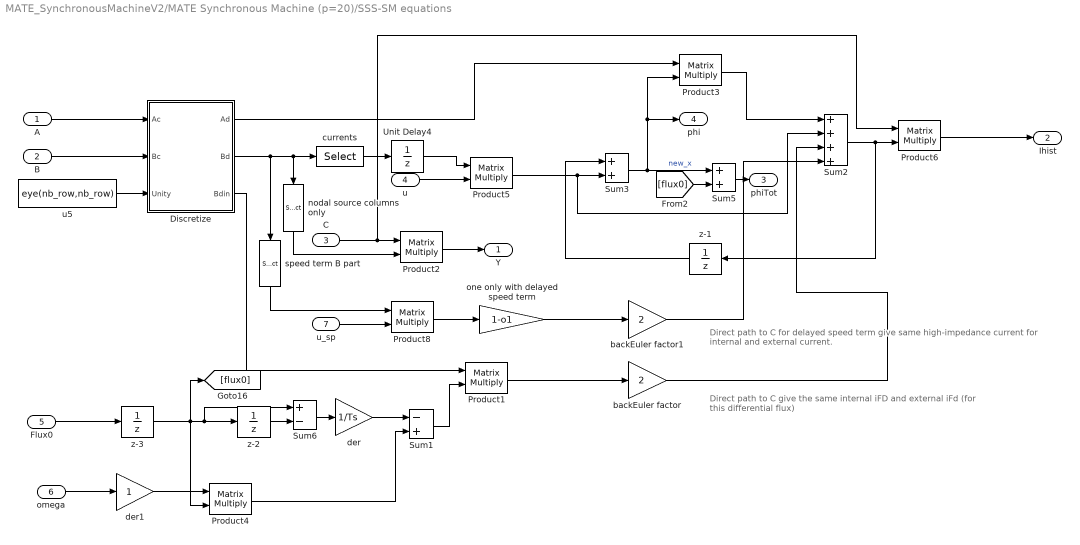
== system MATE_SynchronousMachineV2/MATE Synchronous Machine (p=20)/SSS-SM equations ==
  note: Direct path to C for delayed speed term give same high-impedance current
      | for internal and external current.
  note: Direct path to C give the same internal iFD and external iFd
      | (for this differential flux)
  A : Inport
  B : Inport  Port=2
  C : Inport  Port=3
  u : Inport  Port=4
  Flux0 : Inport  Port=5
  omega : Inport  Port=6
  u_sp : Inport  Port=7
  Discretize : Subsystem
  Product{1..6,8} (7 alike) : Product  Multiplication=Matrix(*)  SaturateOnIntegerOverflow=on  OutDataTypeStr=Inherit: Same as first input
  Sum1 : Sum  Inputs=-+  SaturateOnIntegerOverflow=on
  Sum2 : Sum  Inputs=++++  SaturateOnIntegerOverflow=on
  Sum3 : Sum  SaturateOnIntegerOverflow=on
  Sum5 : Sum  SaturateOnIntegerOverflow=on
  Sum6 : Sum  Inputs=+-  SaturateOnIntegerOverflow=on
  Unit Delay4 : UnitDelay  SampleTime=Ts  HasFrameUpgradeWarning=on
  backEuler factor : Gain  Gain=2  SaturateOnIntegerOverflow=on  OutDataTypeStr=Inherit: Same as input  ParamDataTypeStr=Inherit: Same as input
  backEuler factor1 : Gain  Gain=2  SaturateOnIntegerOverflow=on  OutDataTypeStr=Inherit: Same as input  ParamDataTypeStr=Inherit: Same as input
  currents : Selector  NumberOfDimensions=2  InputPortWidth=3  IndexOptions=Index vector (dialog),Index vector (dialog)  Indices=[1:nb_row],[1 2 3 4]  OutputSizes=1,1
  der : Gain  Gain=1/Ts  SaturateOnIntegerOverflow=on  OutDataTypeStr=Inherit: Same as input  ParamDataTypeStr=Inherit: Same as input
  der1 : Gain  SaturateOnIntegerOverflow=on  OutDataTypeStr=Inherit: Same as input  ParamDataTypeStr=Inherit: Same as input
  nodal source columns only : Selector  NumberOfDimensions=2  InputPortWidth=3  IndexOptions=Index vector (dialog),Index vector (dialog)  Indices=[1:nb_row],[1 2 3 4]  OutputSizes=1,1
  one only with delayed speed term : Gain  Gain=1-o1
  speed term B part : Selector  NumberOfDimensions=2  InputPortWidth=3  IndexOptions=Index vector (dialog),Index vector (dialog)  Indices=[1:nb_row],[5:4+nb_row]  OutputSizes=1,1
  u5 : Constant  Value=eye(nb_row,nb_row)
  z-1 : UnitDelay  InitialCondition=flux_0  SampleTime=Ts  HasFrameUpgradeWarning=on
  z-2 : UnitDelay  SampleTime=Ts  HasFrameUpgradeWarning=on
  z-3 : UnitDelay  SampleTime=Ts  HasFrameUpgradeWarning=on
  Y : Outport  VectorParamsAs1DForOutWhenUnconnected=off
  Ihist : Outport  Port=2  VectorParamsAs1DForOutWhenUnconnected=off
  phiTot : Outport  Port=3  VectorParamsAs1DForOutWhenUnconnected=off
  phi : Outport  Port=4  VectorParamsAs1DForOutWhenUnconnected=off
  wires:
  backEuler factor1/1 -> Sum2/4
  one only with delayed speed term/1 -> backEuler factor1/1
  Product8/1 -> one only with delayed speed term/1
  speed term B part/1 -> Product8/1
  u_sp/1 -> Product8/2
  currents/1 -> Unit Delay4/1
  Unit Delay4/1 -> Product5/1
  backEuler factor/1 -> Sum2/3
  Product1/1 -> backEuler factor/1
  Sum1/1 -> Product1/2
  der1/1 -> Product4/1
  [flux0] -> Sum5/2
  der/1 -> Sum1/1
  Product4/1 -> Sum1/2
  omega/1 -> der1/1
  Discretize/3(Bdin) -> Product1/1
  z-3/1 -> Sum6/1, z-2/1, Product4/2, [flux0]
  Sum6/1 -> der/1
  z-2/1 -> Sum6/2
  Sum5/1 -> phiTot/1
  Flux0/1 -> z-3/1
  Discretize/2(Bd) -> speed term B part/1, currents/1, nodal source columns only/1
  z-1/1 -> Sum3/1
  u/1 -> Product5/2
  Discretize/1(Ad) -> Product3/1
  Sum2/1 -> Product6/2, z-1/1
  Sum3/1 -> phi/1, Product3/2, Sum5/1  "new_x"
  Product3/1 -> Sum2/1
  Product5/1 -> Sum3/2, Sum2/2
  Product6/1 -> Ihist/1
  C/1 -> Product6/1, Product2/1
  B/1 -> Discretize/2(Bc)
  A/1 -> Discretize/1(Ac)
  Product2/1 -> Y/1
  u5/1 -> Discretize/3(Unity)
  nodal source columns only/1 -> Product2/2

== system MATE_SynchronousMachineV2/MATE Synchronous Machine (p=20)/SSS-SM equations zero sequence only ==
  A : Inport
  B : Inport  Port=2
  C : Inport  Port=3
  u : Inport  Port=4
  Discretize : Subsystem
  Product{2..3,5..6} (4 alike) : Product  Multiplication=Matrix(*)  SaturateOnIntegerOverflow=on  OutDataTypeStr=Inherit: Same as first input
  Sum2 : Sum  SaturateOnIntegerOverflow=on
  Sum3 : Sum  SaturateOnIntegerOverflow=on
  u5 : Constant
  z-1 : UnitDelay  SampleTime=Ts  HasFrameUpgradeWarning=on
  Y0 : Outport  VectorParamsAs1DForOutWhenUnconnected=off
  Ihist0 : Outport  Port=2  VectorParamsAs1DForOutWhenUnconnected=off
  phi0 : Outport  Port=3  VectorParamsAs1DForOutWhenUnconnected=off
  wires:
  Discretize/2(Bd) -> Product2/2, Product5/1
  z-1/1 -> Sum3/1
  u/1 -> Product5/2
  Discretize/1(Ad) -> Product3/1
  Sum2/1 -> Product6/2, z-1/1
  Sum3/1 -> phi0/1, Product3/2  "new_x"
  Product3/1 -> Sum2/1
  Product5/1 -> Sum3/2, Sum2/2
  Product6/1 -> Ihist0/1
  C/1 -> Product2/1, Product6/1
  B/1 -> Discretize/2(Bc)
  A/1 -> Discretize/1(Ac)
  Product2/1 -> Y0/1
  u5/1 -> Discretize/3(Unity)

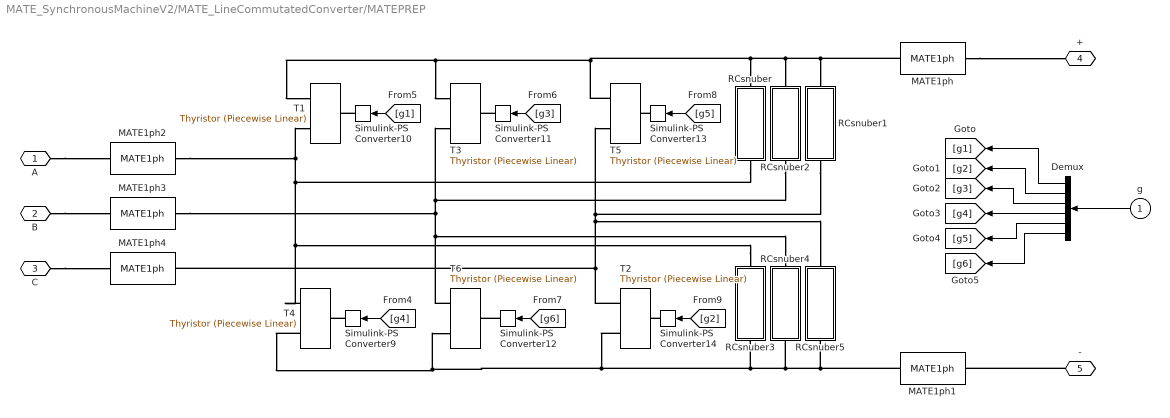
== system MATE_SynchronousMachineV2/MATE_LineCommutatedConverter/MATEPREP ==
  g : Inport
  Demux : Demux  Outputs=6
  MATE1ph : simetran/MATE1ph  bn=4  conty=Single-Phase  it=auto  Rse=1e-4  Rsh=1e9
      settings: AttributesFormatString=# %<bn>
  MATE1ph1 : simetran/MATE1ph  bn=5  conty=Single-Phase  it=auto  Rse=1e-4  Rsh=1e9
      settings: AttributesFormatString=# %<bn>
  MATE1ph2 : simetran/MATE1ph  bn=1  conty=Single-Phase  it=auto  Rse=1e-4  Rsh=1e9
      settings: AttributesFormatString=# %<bn>
  MATE1ph3 : simetran/MATE1ph  bn=2  conty=Single-Phase  it=auto  Rse=1e-4  Rsh=1e9
      settings: AttributesFormatString=# %<bn>
  MATE1ph4 : simetran/MATE1ph  bn=3  conty=Single-Phase  it=auto  Rse=1e-4  Rsh=1e9
      settings: AttributesFormatString=# %<bn>
  RCsnuber : Subsystem
  RCsnuber1 : Subsystem
  RCsnuber2 : Subsystem
  RCsnuber3 : Subsystem
  RCsnuber4 : Subsystem
  RCsnuber5 : Subsystem
  Simulink-PS Converter{9..14} (6 alike) : nesl_utility/Simulink-PS Converter  PhysicalDomain=network_engine_domain  SubClassName=ps_input  LeftPortType=input  RightPortType=output  PseudoPeriodic=off  Frequencies=[]  NoiseDistribution=none  NoiseParameters=[]  Unit=1  AffineConversion=off  FilteringAndDerivatives=provide  SimscapeFilterOrder=1  InputFilterTimeConstant=0.001  UdotUserProvided=0
  T{1..6} (6 alike) : ee_lib/Semiconductors & Converters/Thyristor (Piecewise Linear)  port_option=ee.enum.controlport.ps  Vf=0.8 V  Ron=0.001 Ohm  Goff=1e-5 1/Ohm  Vgt=0.5 V  Ih=1 A  diode_param=ee.enum.semiconductors.protectionDiode.external  diode_Vf=0.8 V  diode_Ron=0.001 Ohm  diode_Goff=1e-5 1/Ohm  diode_C=50e-9 F  diode_iRM=-235 A  diode_iF=300 A  diode_idot=-50 A/us  diode_trr_param=ee.enum.converters.diodetrr.trr_factor  diode_trr_factor=3  diode_trr=15 us  diode_Qrr=1500 s*uA  iak_specify=off  iak_priority=None  iak=0 A  iak_nominal_specify=off  iak_nominal_value=1  iak_nominal_unit=A  vak_specify=off  vak_priority=None  vak=0 V  vak_nominal_specify=off  vak_nominal_value=1  vak_nominal_unit=V  vgk_specify=off  vgk_priority=None  vgk=0 V  vgk_nominal_specify=off  vgk_nominal_value=1  vgk_nominal_unit=V  thermal_loss_option=ee.enum.converters.thermalLossOption.constantvalues  Von_data=[0, .1, .6, .8, 1, 1.3, 1.6, 2, 2.4; 0, .1, .7, 1, 1.2, 1.5, 1.9, 2.4, 2.8] V  Tj=[298.15, 398.15] K  Iout_data=[0, .1, 1, 5, 10, 20, 40, 70, 100] A  Eon_data=[0, .0024, .024, .12, .2, .48, 1.04, 2.16, 3.24; 0, .003, .03, .15, .25, .6, 1.3, 2.7, 4.05] * 1e-3 J  Tj_loss=[298.15, 398.15] K  Iout_data_loss=[0, .1, 1, 5, 10, 20, 40, 70, 100] A  Eon_scalar=22.86e-3 J  Eoff_natural_commutation=10e-3 J  Voff=300 V  Iout_scalar=600 A  onCurrentMeasDelay=1e-4 s  diodeModelType=ee.enum.converters.diodeModelType.pwl  diodeTableType=ee.enum.diode.tableType.IfMat  diode_IfMat=[.07, .12, .19, 1.75, 4.24, 7.32, 11.2; .16, .3, .72, 2.14, 4.02, 6.35, 9.12] A  diode_VfMat=[.9, 1.15, 1.25, 1.5, 1.75, 2.17, 2.6, 2.85; .58, .68, .75, 1.1, 1.38, 1.77, 2.27, 2.7] V  diode_TjVec=[25, 125] degC  diode_VfVec=[.5, .7, .9, 1.3, 1.7, 2.1, 2.5] V  diode_IfVec=[.1, .2, .5, 1, 2, 4, 7, 10] A  diode_rec_loss_model=ee.enum.diode.reverseRecoveryModel.fixed  diode_ErecVal=0 J  diode_scaleWithIandV=true  diode_ErecMat=zeros(2, 3) J  diode_TjrecVec=[298.15, 398.15] K  diode_IfrecVec=[.1, 1, 10] A  diode_IrecVal=10 A  diode_VrecVal=10 V  diode_tFilter=1 / 1000 / 100 s  thermal_network_parameterization=ee.enum.thermalNetworkTopology.external  Rth=[.08, .5] K/W  Rth_Cauer=[.08, .1, .5] K/W  Rth_Foster=[.08, .14, .22, .16] K/W  thermal_mass_parameterization=ee.enum.thermalNetwork.timeconstant  thermal_mass=[.01, .5] J/K  thermal_mass_Cauer=[.01, .1, .5] J/K  thermal_mass_Foster=[.001, .005, .05, .5] J/K  thermal_time_constant=[.001, .2] s  thermal_time_constant_Cauer=[.001, .1, .2] s  thermal_time_constant_Foster=[7e-05, .0007, .01, .08] s  thermal_mass_initial_temperatures=[25, 25] degC  thermal_mass_initial_temperatures_Cauer=[25, 25, 25] degC  junction_thermal_mass=0.01 J/K  Tvec_initial_Foster=[25, 25, 25, 25] degC  junction_temperature_specify=off  junction_temperature_priority=None  junction_temperature=25 degC  junction_temperature_nominal_specify=off  junction_temperature_nominal_value=1  junction_temperature_nominal_unit=degC  Qj_specify=off  Qj_priority=None  Qj=0 W  Qj_nominal_specify=off  Qj_nominal_value=1  Qj_nominal_unit=W  accumulatedSwitchingLosses_specify=off  accumulatedSwitchingLosses_priority=None  accumulatedSwitchingLosses=0 J
      settings: InternalSimscapePortConfiguration="{\"Bottom\":[],\"Left\":[{\"id\":\"G\",\"label\":\"\",\"type\":\"input\"}],\"Right\":[{\"id\":\"A\",\"label\":\"\",\"type\":\"foundation.electrical.electrical\"},{\"id\":\"K\",\"label\":\"\",\"type\":\"foundation.electrical.electrical\"}],\"Top\":[]}"
  A : PMIOPort  Side=Left
  B : PMIOPort  Port=2  Side=Left
  C : PMIOPort  Port=3  Side=Left
  + : PMIOPort  Port=4  Side=Right
  - : PMIOPort  Port=5  Side=Right
  wires:
  Demux/5 -> [g5]
  Demux/6 -> [g6]
  Demux/4 -> [g4]
  Demux/3 -> [g3]
  Demux/2 -> [g2]
  Demux/1 -> [g1]
  g/1 -> Demux/1
  [g4] -> Simulink-PS Converter9/1
  [g1] -> Simulink-PS Converter10/1
  [g3] -> Simulink-PS Converter11/1
  [g6] -> Simulink-PS Converter12/1
  [g5] -> Simulink-PS Converter13/1
  [g2] -> Simulink-PS Converter14/1
  connections:
  RCsnuber3/LConn1 -- T4/RConn2 -- RCsnuber/RConn1 -- MATE1ph2/RConn1 -- T1/RConn1
  MATE1ph3/RConn1 -- RCsnuber2/RConn1 -- T3/RConn1 -- T6/RConn2 -- RCsnuber4/LConn1
  RCsnuber1/RConn1 -- T5/RConn1 -- T2/RConn2 -- MATE1ph4/RConn1 -- RCsnuber5/LConn1
  RCsnuber4/RConn1 -- MATE1ph1/RConn1 -- RCsnuber5/RConn1 -- T2/RConn1 -- T6/RConn1 -- T4/RConn1 -- RCsnuber3/RConn1
  MATE1ph/RConn1 -- T1/RConn2 -- T3/RConn2 -- T5/RConn2 -- RCsnuber/LConn1 -- RCsnuber2/LConn1 -- RCsnuber1/LConn1
  -/RConn1 -- MATE1ph1/LConn1
  A/RConn1 -- MATE1ph2/LConn1
  B/RConn1 -- MATE1ph3/LConn1
  C/RConn1 -- MATE1ph4/LConn1
  Simulink-PS Converter9/RConn1 -- T4/LConn1
  Simulink-PS Converter10/RConn1 -- T1/LConn1
  Simulink-PS Converter11/RConn1 -- T3/LConn1
  Simulink-PS Converter12/RConn1 -- T6/LConn1
  Simulink-PS Converter13/RConn1 -- T5/LConn1
  Simulink-PS Converter14/RConn1 -- T2/LConn1
  MATE1ph/LConn1 -- +/RConn1
